simulink model "AM_Mod_coherent"  (R2015b)
settings: Solver=ode3  StartTime=0.0  StopTime=10  FixedStep=0.000001  RelTol=1e-3
undefined symbols (not defined in the file): n
libraries: dsparch4 x1
settings Model: Creator=Ishraque  LastModifiedBy=cwang135
settings DataIOCC: SaveFormat=Array
settings DebuggingCC: SolverPrmCheckMsg=warning
settings HardwareCC: ProdBitPerPointer=32  ProdLargestAtomicFloat=None  ProdIntDivRoundTo=Undefined  ProdEndianess=Unspecified  ProdWordSize=32  ProdHWDeviceType=32-bit Generic
settings GRTTargetCC: GeneratePreprocessorConditionals=Disable all
settings ConfigComp: CovModelRefEnable=Off  CovSFcnEnable=off

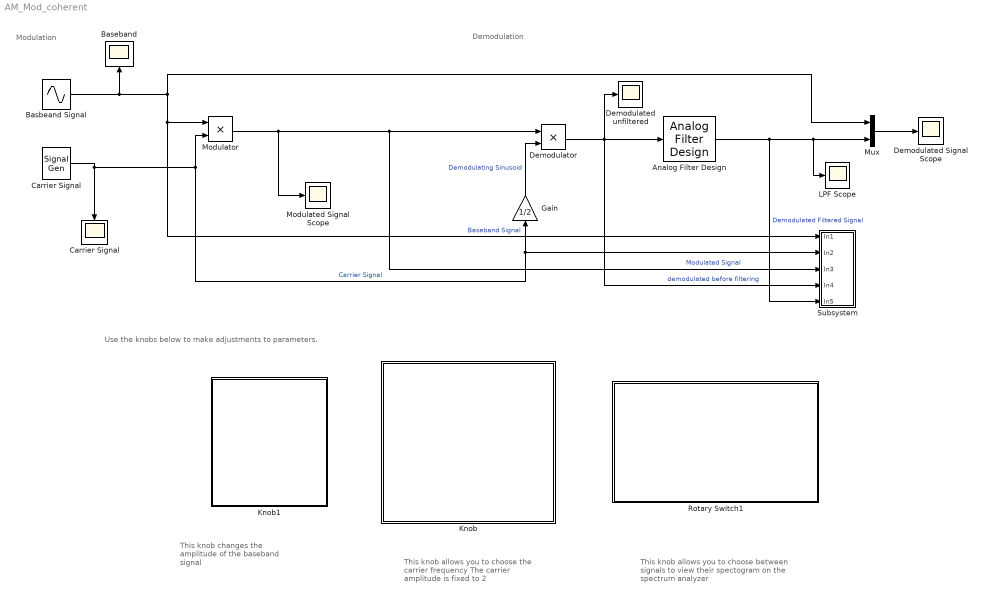
== system AM_Mod_coherent ==
  note: Demodulation
  note: Modulation
  note: Use the knobs below to make adjustments to parameters.
  note: This knob allows you to choose between
      | signals to view their spectogram on the
      | spectrum analyzer
  note: This knob allows you
      | to choose the carrier frequency
      | The carrier amplitude is fixed to 2
  note: This knob changes the
      | amplitude of the baseband
      | signal
  Analog Filter Design : dsparch4/Analog Filter Design  method=Butterworth  filttype=Lowpass  N=n  Wlo=cutoff  Whi=80  Rp=2  Rs=40
  "Basbeand Signal " : Sin  Frequency=2*pi*2000  SampleTime=0
  Baseband : Scope
  Carrier Signal : SignalGenerator  Amplitude=2  Frequency=20000
  "Carrier Signal " : Scope
  Demodulated Signal Scope : Scope
  Demodulated unfiltered : Scope
  Demodulator : Product
  Gain : Gain  Gain=1/2
  Knob : Subsystem  DialogController=hmiCreateDDGDialog  IsWebBlock=on  mask(MWDashboardBlock){webBlockId=54b8352b-1b71-4207-b929-ffcb71418978, webBlockType=continuousknob, ShowInLibBrowser=on, ShowInitialText=on, HMISrcModelName=AM_Mod_coherent}
      mask prompts: webBlockId "WebBlock Id"; webBlockType "WebBlock Type"; HMISrcModelName "Source Model"
      mask Help: helpview([docroot '/mapfiles/simulink.map'], 'hmi_knob')
      mask Display:
      | if strcmp(get_param(bdroot(gcb),'BlockDiagramType'), 'library')
      |     image([(matlabroot) '/toolbox/simulink/hmi/icons/ContinuousKnob.png']);
      | end
  Knob1 : Subsystem  DialogController=hmiCreateDDGDialog  IsWebBlock=on  mask(MWDashboardBlock){webBlockId=b6505c6d-90bc-4c35-a436-f01c23a38622, webBlockType=continuousknob, ShowInLibBrowser=on, ShowInitialText=on, HMISrcModelName=AM_Mod_coherent}
      mask prompts: webBlockId "WebBlock Id"; webBlockType "WebBlock Type"; HMISrcModelName "Source Model"
      mask Help: helpview([docroot '/mapfiles/simulink.map'], 'hmi_knob')
      mask Display:
      | if strcmp(get_param(bdroot(gcb),'BlockDiagramType'), 'library')
      |     image([(matlabroot) '/toolbox/simulink/hmi/icons/ContinuousKnob.png']);
      | end
  LPF Scope : Scope
  Modulated Signal Scope : Scope
  Modulator : Product
  Mux : Mux  Inputs=2
  Rotary Switch1 : Subsystem  DialogController=hmiCreateDDGDialog  IsWebBlock=on  mask(MWDashboardBlock){webBlockId=534c7ef2-1674-4c23-9e54-a44f8668b583, webBlockType=discreteknob, ShowInLibBrowser=on, ShowInitialText=on, HMISrcModelName=AM_Mod_coherent}
      mask prompts: webBlockId "WebBlock Id"; webBlockType "WebBlock Type"; HMISrcModelName "Source Model"
      mask Help: helpview([docroot '/mapfiles/simulink.map'], 'hmi_rotary_switch')
      mask Display:
      | model = bdroot(gcb);
      | if strcmp(get_param(model,'BlockDiagramType'), 'library')
      |     image([(matlabroot) '/toolbox/simulink/hmi/icons/DiscreteKnob.png']);
      | end
  Subsystem : Subsystem
  wires:
  Modulator/1 -> Subsystem/3(In3), Demodulator/1, Modulated Signal Scope/1  "Modulated Signal"
  Demodulator/1 -> Subsystem/4(In4), Analog Filter Design/1, Demodulated unfiltered/1  "demodulated before filtering"
  Analog Filter Design/1 -> Mux/2, LPF Scope/1, Subsystem/5(In5)  "Demodulated Filtered Signal"
  Carrier Signal/1 -> Gain/1, Subsystem/2(In2), Modulator/2, "Carrier Signal "/1  "Carrier Signal"
  "Basbeand Signal "/1 -> Baseband/1, Mux/1, Modulator/1, Subsystem/1(In1)  "Baseband Signal"
  Gain/1 -> Demodulator/2  "Demodulating Sinusoid"
  Mux/1 -> Demodulated Signal Scope/1

== system AM_Mod_coherent/Knob ==

== system AM_Mod_coherent/Knob1 ==

== system AM_Mod_coherent/Rotary Switch1 ==

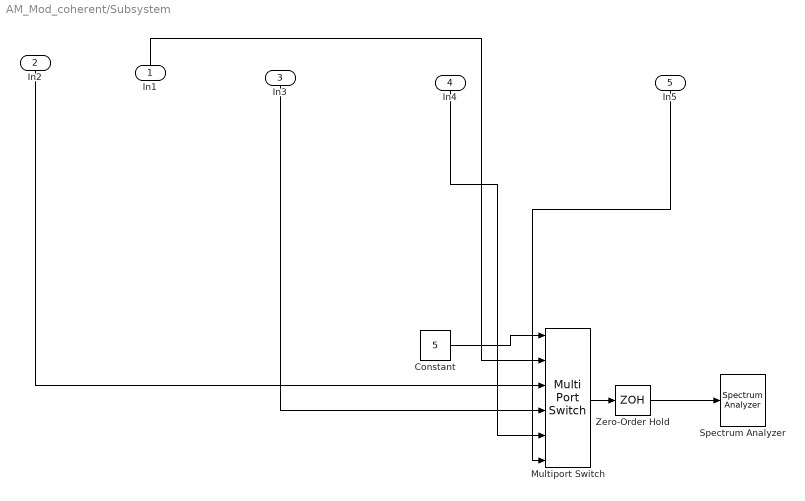
== system AM_Mod_coherent/Subsystem ==
  In1 : Inport
  In2 : Inport  Port=2
  In3 : Inport  Port=3
  In4 : Inport  Port=4
  In5 : Inport  Port=5
  Constant : Constant  Value=5
  Multiport Switch : MultiPortSwitch  Inputs=5
  Spectrum Analyzer : SpectrumAnalyzer
  Zero-Order Hold : ZeroOrderHold  SampleTime=1e-5
  wires:
  Zero-Order Hold/1 -> Spectrum Analyzer/1
  Multiport Switch/1 -> Zero-Order Hold/1
  Constant/1 -> Multiport Switch/1
  In1/1 -> Multiport Switch/2
  In2/1 -> Multiport Switch/3
  In4/1 -> Multiport Switch/5
  In5/1 -> Multiport Switch/6
  In3/1 -> Multiport Switch/4
